simulink library "inp"  (R2021b)
settings: Solver=VariableStepAuto  StartTime=0.0  StopTime=10.0  RelTol=1e-3
undefined symbols (not defined in the file): C_TASK_5MS_S, FALSE, KINP_AcoreReadyToSlp_flg_ovrdflg, KINP_AcoreReadyToSlp_flg_ovrdval, KINP_AllowMovThd_OTA_enum_ovrdflg, KINP_AllowMovThd_OTA_enum_ovrdval, KINP_APSAngleTarget_Deg_ovrdflg, KINP_APSAngleTarget_Deg_ovrdval, KINP_APSDecReq_mps2_ovrdflg, KINP_APSDecReq_mps2_ovrdval, KINP_APSDecReqA_flg_ovrdflg, KINP_APSDecReqA_flg_ovrdval, KINP_APSDFLL_cm_ovrdflg, KINP_APSDFLL_cm_ovrdval, KINP_APSDFLR_cm_ovrdflg, KINP_APSDFLR_cm_ovrdval, KINP_APSDRLL_cm_ovrdflg, KINP_APSDRLL_cm_ovrdval, KINP_APSDRLR_cm_ovrdflg, KINP_APSDRLR_cm_ovrdval, KINP_APSExitCondition_enum_ovrdflg, KINP_APSExitCondition_enum_ovrdval, KINP_APSHWVer_enum_ovrdflg, KINP_APSHWVer_enum_ovrdval, KINP_APSProgressPCT_pct_ovrdflg, KINP_APSProgressPCT_pct_ovrdval, KINP_APSPwrReq_enum_ovrdflg, KINP_APSPwrReq_enum_ovrdval, KINP_APSReq_enum_ovrdflg, KINP_APSReq_enum_ovrdval, KINP_APSRQDisplay_enum_ovrdflg, KINP_APSRQDisplay_enum_ovrdval, KINP_APSRqEPASCtrl_flg_ovrdflg, KINP_APSRqEPASCtrl_flg_ovrdval, KINP_APSShiftPosnReq_enum_ovrdval, KINP_APSShiftPosnReq_enum_ovrflg, KINP_APSSpeedCMD_kph_ovrdval, KINP_APSSpeedCMD_kph_ovrflg, KINP_APSStaSystem_enum_ovrdflg, KINP_APSStaSystem_enum_ovrdval, KINP_APSSWVer_enum_ovrdflg, KINP_APSSWVer_enum_ovrdval, KINP_APSVMCReqA_flg_ovrdval, KINP_APSVMCReqA_flg_ovrflg, KINP_APSVRqEPASCtrl_flg_ovrdflg, KINP_APSVRqEPASCtrl_flg_ovrdval, KINP_AuxBattVolmV_mV_ovrdflg, KINP_AuxBattVolmV_mV_ovrdval, KINP_CAASSta_enum_ovrdflg, KINP_CAASSta_enum_ovrdval, KINP_CAASVMCReqA_flg_ovrdval, KINP_CAASVMCReqA_flg_ovrflg, KINP_CAN1BusOff_flg_ovrdflg, KINP_CAN1BusOff_flg_ovrdval, KINP_CAN2BusOff_flg_ovrdflg, KINP_CAN2BusOff_flg_ovrdval, KINP_CAN3BusOff_flg_ovrdflg, KINP_CAN3BusOff_flg_ovrdval, KINP_CAN4BusOff_flg_ovrdflg, KINP_CAN4BusOff_flg_ovrdval ... (+152)
libraries: FVT_lib x1037, hcu_lib x1
(part 12 of 34)

== system inp/INP/SYS/Subsystem ==
  In1 : Inport
  Constant : Constant  Value=KINP_AuxBattVolmV_mV_ovrdflg
  Constant1 : Constant  Value=KINP_AuxBattVolmV_mV_ovrdval
  Switch : Switch  Criteria=u2 > Threshold
  Out1 : Outport
  wires:
  Constant1/1 -> Switch/1
  Constant/1 -> Switch/2
  In1/1 -> Switch/3
  Switch/1 -> Out1/1

== system inp/INP/SYS/Subsystem1 ==
  In1 : Inport
  Constant : Constant  Value=KINP_NetworkReqCalled_flg_ovrdflg
  Constant1 : Constant  Value=KINP_NetworkReqCalled_flg_ovrdval
  Switch : Switch  Criteria=u2 > Threshold
  Out1 : Outport
  wires:
  Constant1/1 -> Switch/1
  Constant/1 -> Switch/2
  In1/1 -> Switch/3
  Switch/1 -> Out1/1

== system inp/INP/SYS/Subsystem10 ==
  In1 : Inport
  Constant : Constant  Value=KINP_CAN3BusOff_flg_ovrdflg
  Constant1 : Constant  Value=KINP_CAN3BusOff_flg_ovrdval
  Switch : Switch  Criteria=u2 > Threshold
  Out1 : Outport
  wires:
  Constant1/1 -> Switch/1
  Constant/1 -> Switch/2
  In1/1 -> Switch/3
  Switch/1 -> Out1/1

== system inp/INP/SYS/Subsystem11 ==
  In1 : Inport
  Constant : Constant  Value=KINP_CAN6BusOff_flg_ovrdflg
  Constant1 : Constant  Value=KINP_CAN6BusOff_flg_ovrdval
  Switch : Switch  Criteria=u2 > Threshold
  Out1 : Outport
  wires:
  Switch/1 -> Out1/1
  In1/1 -> Switch/3
  Constant/1 -> Switch/2
  Constant1/1 -> Switch/1

== system inp/INP/SYS/Subsystem12 ==
  In1 : Inport
  Constant : Constant  Value=KINP_CAN4BusOff_flg_ovrdflg
  Constant1 : Constant  Value=KINP_CAN4BusOff_flg_ovrdval
  Switch : Switch  Criteria=u2 > Threshold
  Out1 : Outport
  wires:
  Switch/1 -> Out1/1
  In1/1 -> Switch/3
  Constant/1 -> Switch/2
  Constant1/1 -> Switch/1

== system inp/INP/SYS/Subsystem13 ==
  In1 : Inport
  Constant : Constant  Value=KINP_CAN5BusOff_flg_ovrdflg
  Constant1 : Constant  Value=KINP_CAN5BusOff_flg_ovrdval
  Switch : Switch  Criteria=u2 > Threshold
  Out1 : Outport
  wires:
  Constant1/1 -> Switch/1
  Constant/1 -> Switch/2
  In1/1 -> Switch/3
  Switch/1 -> Out1/1

== system inp/INP/SYS/Subsystem2 ==
  In1 : Inport
  Constant : Constant  Value=KINP_Pedal1Ref5V_V_ovrdflg
  Constant1 : Constant  Value=KINP_Pedal1Ref5V_V_ovrdval
  Switch : Switch  Criteria=u2 > Threshold
  Out1 : Outport
  wires:
  Switch/1 -> Out1/1
  In1/1 -> Switch/3
  Constant/1 -> Switch/2
  Constant1/1 -> Switch/1

== system inp/INP/SYS/Subsystem3 ==
  In1 : Inport
  Constant : Constant  Value=KINP_Pedal2Ref5V_V_ovrdflg
  Constant1 : Constant  Value=KINP_Pedal2Ref5V_V_ovrdval
  Switch : Switch  Criteria=u2 > Threshold
  Out1 : Outport
  wires:
  Constant1/1 -> Switch/1
  Constant/1 -> Switch/2
  In1/1 -> Switch/3
  Switch/1 -> Out1/1

== system inp/INP/SYS/Subsystem4 ==
  In1 : Inport
  Constant : Constant  Value=KINP_PwrReq_OTA_enum_ovrdval
  Constant1 : Constant  Value=KINP_PwrReq_OTA_enum_ovrdflg
  Switch : Switch  Criteria=u2 ~= 0
  Out1 : Outport
  wires:
  Constant1/1 -> Switch/2
  Constant/1 -> Switch/1
  In1/1 -> Switch/3
  Switch/1 -> Out1/1

== system inp/INP/SYS/Subsystem5 ==
  In1 : Inport
  Constant : Constant  Value=KINP_AllowMovThd_OTA_enum_ovrdval
  Constant1 : Constant  Value=KINP_AllowMovThd_OTA_enum_ovrdflg
  Switch : Switch  Criteria=u2 ~= 0
  Out1 : Outport
  wires:
  Switch/1 -> Out1/1
  In1/1 -> Switch/3
  Constant/1 -> Switch/1
  Constant1/1 -> Switch/2

== system inp/INP/SYS/Subsystem6 ==
  In1 : Inport
  Constant : Constant  Value=KINP_EvccAplusPwrUpReq_flg_ovrdval
  Constant1 : Constant  Value=KINP_EvccAplusPwrUpReq_flg_ovrdflg
  Switch : Switch  Criteria=u2 ~= 0
  Out1 : Outport
  wires:
  Constant1/1 -> Switch/2
  Constant/1 -> Switch/1
  In1/1 -> Switch/3
  Switch/1 -> Out1/1

== system inp/INP/SYS/Subsystem7 ==
  In1 : Inport
  Constant : Constant  Value=KINP_AcoreReadyToSlp_flg_ovrdval
  Constant1 : Constant  Value=KINP_AcoreReadyToSlp_flg_ovrdflg
  Switch : Switch  Criteria=u2 ~= 0
  Out1 : Outport
  wires:
  Switch/1 -> Out1/1
  In1/1 -> Switch/3
  Constant/1 -> Switch/1
  Constant1/1 -> Switch/2

== system inp/INP/SYS/Subsystem8 ==
  In1 : Inport
  Constant : Constant  Value=KINP_CAN1BusOff_flg_ovrdflg
  Constant1 : Constant  Value=KINP_CAN1BusOff_flg_ovrdval
  Switch : Switch  Criteria=u2 > Threshold
  Out1 : Outport
  wires:
  Constant1/1 -> Switch/1
  Constant/1 -> Switch/2
  In1/1 -> Switch/3
  Switch/1 -> Out1/1

== system inp/INP/SYS/Subsystem9 ==
  In1 : Inport
  Constant : Constant  Value=KINP_CAN2BusOff_flg_ovrdflg
  Constant1 : Constant  Value=KINP_CAN2BusOff_flg_ovrdval
  Switch : Switch  Criteria=u2 > Threshold
  Out1 : Outport
  wires:
  Switch/1 -> Out1/1
  In1/1 -> Switch/3
  Constant/1 -> Switch/2
  Constant1/1 -> Switch/1

== system inp/INP/TPMS/Subsystem ==
  In1 : Inport
  Constant : Constant  Value=KINP_TPMSDataIn_flg_ovrdval
  Constant1 : Constant  Value=KINP_TPMSDataIn_flg_ovrdflg
  Switch : Switch  Criteria=u2 ~= 0
  Out1 : Outport
  wires:
  Switch/1 -> Out1/1
  In1/1 -> Switch/3
  Constant/1 -> Switch/1
  Constant1/1 -> Switch/2

== system inp/INP/TPMS/Subsystem1 ==
  In1 : Inport
  Constant : Constant  Value=KINP_TPMSID_raw_ovrdflg
  Constant1 : Constant  Value=KINP_TPMSID_raw_ovrdval
  Switch : Switch  Criteria=u2 ~= 0
  Out1 : Outport
  wires:
  Constant/1 -> Switch/2
  Constant1/1 -> Switch/1
  Switch/1 -> Out1/1
  In1/1 -> Switch/3

== system inp/INP/TPMS/Subsystem10 ==
  In1 : Inport
  Constant : Constant  Value=KINP_TPMSStorge_flg_ovrflg
  Constant1 : Constant  Value=KINP_TPMSStorge_flg_ovrdval
  Switch : Switch  Criteria=u2 ~= 0
  Out1 : Outport
  wires:
  Constant1/1 -> Switch/1
  Constant/1 -> Switch/2
  In1/1 -> Switch/3
  Switch/1 -> Out1/1

== system inp/INP/TPMS/Subsystem11 ==
  In1 : Inport
  Constant : Constant  Value=KINP_LFID_raw_ovrflg
  Constant1 : Constant  Value=KINP_LFID_raw_ovrdval
  Switch : Switch  Criteria=u2 ~= 0
  Out1 : Outport
  wires:
  Switch/1 -> Out1/1
  In1/1 -> Switch/3
  Constant/1 -> Switch/2
  Constant1/1 -> Switch/1

== system inp/INP/TPMS/Subsystem12 ==
  In1 : Inport
  Constant : Constant  Value=KINP_RFID_raw_ovrdval
  Constant1 : Constant  Value=KINP_RFID_raw_ovrdval
  Switch : Switch  Criteria=u2 ~= 0
  Out1 : Outport
  wires:
  Constant1/1 -> Switch/1
  Constant/1 -> Switch/2
  In1/1 -> Switch/3
  Switch/1 -> Out1/1

== system inp/INP/TPMS/Subsystem13 ==
  In1 : Inport
  Constant : Constant  Value=KINP_LRID_raw_ovrdval
  Constant1 : Constant  Value=KINP_LRID_raw_ovrdval
  Switch : Switch  Criteria=u2 ~= 0
  Out1 : Outport
  wires:
  Switch/1 -> Out1/1
  In1/1 -> Switch/3
  Constant/1 -> Switch/2
  Constant1/1 -> Switch/1

== system inp/INP/TPMS/Subsystem14 ==
  In1 : Inport
  Constant : Constant  Value=KINP_RRID_raw_ovrdval
  Constant1 : Constant  Value=KINP_RRID_raw_ovrdval
  Switch : Switch  Criteria=u2 ~= 0
  Out1 : Outport
  wires:
  Constant1/1 -> Switch/1
  Constant/1 -> Switch/2
  In1/1 -> Switch/3
  Switch/1 -> Out1/1

== system inp/INP/TPMS/Subsystem2 ==
  In1 : Inport
  Constant : Constant  Value=KINP_TPMSPressure_raw_ovrdflg
  Constant1 : Constant  Value=KINP_TPMSPressure_raw_ovrdval
  Switch : Switch  Criteria=u2 ~= 0
  Out1 : Outport
  wires:
  Constant/1 -> Switch/2
  Constant1/1 -> Switch/1
  Switch/1 -> Out1/1
  In1/1 -> Switch/3

== system inp/INP/TPMS/Subsystem3 ==
  In1 : Inport
  Constant : Constant  Value=KINP_TPMSTemp_raw_ovrdflg
  Constant1 : Constant  Value=KINP_TPMSTemp_raw_ovrdval
  Switch : Switch  Criteria=u2 ~= 0
  Out1 : Outport
  wires:
  Constant/1 -> Switch/2
  Constant1/1 -> Switch/1
  Switch/1 -> Out1/1
  In1/1 -> Switch/3

== system inp/INP/TPMS/Subsystem4 ==
  In1 : Inport
  Constant : Constant  Value=KINP_TPMSSta_enum_ovrdflg
  Constant1 : Constant  Value=KINP_TPMSSta_enum_ovrdval
  Switch : Switch  Criteria=u2 ~= 0
  Out1 : Outport
  wires:
  Constant/1 -> Switch/2
  Constant1/1 -> Switch/1
  Switch/1 -> Out1/1
  In1/1 -> Switch/3

== system inp/INP/TPMS/Subsystem5 ==
  In1 : Inport
  Constant : Constant  Value=KINP_TPMSPressureMi_raw_ovrdflg
  Constant1 : Constant  Value=KINP_TPMSPressureMi_raw_ovrdval
  Switch : Switch  Criteria=u2 ~= 0
  Out1 : Outport
  wires:
  Constant/1 -> Switch/2
  Constant1/1 -> Switch/1
  Switch/1 -> Out1/1
  In1/1 -> Switch/3

== system inp/INP/TPMS/Subsystem6 ==
  In1 : Inport
  Constant : Constant  Value=KINP_TPMSCRC_crc_ovrdflg
  Constant1 : Constant  Value=KINP_TPMSCRC_crc_ovrdval
  Switch : Switch  Criteria=u2 ~= 0
  Out1 : Outport
  wires:
  Constant/1 -> Switch/2
  Constant1/1 -> Switch/1
  Switch/1 -> Out1/1
  In1/1 -> Switch/3

== system inp/INP/TPMS/Subsystem7 ==
  In1 : Inport
  Constant : Constant  Value=KINP_TPMSCRCCalc_crc_ovrdflg
  Constant1 : Constant  Value=KINP_TPMSCRCCalc_crc_ovrdval
  Switch : Switch  Criteria=u2 ~= 0
  Out1 : Outport
  wires:
  Constant/1 -> Switch/2
  Constant1/1 -> Switch/1
  Switch/1 -> Out1/1
  In1/1 -> Switch/3

== system inp/INP/TPMS/Subsystem8 ==
  In1 : Inport
  Constant : Constant  Value=KINP_TPMSFAT_flg_ovrflg
  Constant1 : Constant  Value=KINP_TPMSFAT_flg_ovrdval
  Switch : Switch  Criteria=u2 ~= 0
  Out1 : Outport
  wires:
  Switch/1 -> Out1/1
  In1/1 -> Switch/3
  Constant1/1 -> Switch/1
  Constant/1 -> Switch/2

== system inp/INP/TPMS/Subsystem9 ==
  In1 : Inport
  Constant : Constant  Value=KINP_TPMSBattLow_flg_ovrflg
  Constant1 : Constant  Value=KINP_TPMSBattLow_flg_ovrdval
  Switch : Switch  Criteria=u2 ~= 0
  Out1 : Outport
  wires:
  Switch/1 -> Out1/1
  In1/1 -> Switch/3
  Constant/1 -> Switch/2
  Constant1/1 -> Switch/1

== system inp/INP/CAN1/SignalCheck/ABM1 ==
  BHAL_outputs : Inport
  inp_CanValid_bus : Inport  Port=2
  ABM1CSErr : FVT_lib/inp/can_signal_template  SystemSampleTime=-1  VariantActivationTime=update diagram  Latency=0  AutoFrameSizeCalculation=off
      link override defval: Value=KINP_ABM1CSErr_flg_defval
      link override ovrdflg: Value=KINP_ABM1CSErr_flg_ovrdflg
      link override ovrdval: Value=KINP_ABM1CSErr_flg_ovrdval
  ABM1RCErr : FVT_lib/inp/can_signal_template  SystemSampleTime=-1  VariantActivationTime=update diagram  Latency=0  AutoFrameSizeCalculation=off
      link override defval: Value=KINP_ABM1RCErr_flg_defval
      link override ovrdflg: Value=KINP_ABM1RCErr_flg_ovrdflg
      link override ovrdval: Value=KINP_ABM1RCErr_flg_ovrdval
  ABMPassengerODSSta : FVT_lib/inp/can_signal_template  SystemSampleTime=-1  VariantActivationTime=update diagram  Latency=0  AutoFrameSizeCalculation=off
      link override defval: Value=KINP_ABMPassengerODSSta_flg_defval
      link override ovrdflg: Value=KINP_ABMPassengerODSSta_flg_ovrdflg
      link override ovrdval: Value=KINP_ABMPassengerODSSta_flg_ovrdval
  ABMRearPassengerCTRODSSta : FVT_lib/inp/can_signal_template  SystemSampleTime=-1  VariantActivationTime=update diagram  Latency=0  AutoFrameSizeCalculation=off
      link override defval: Value=KINP_ABMRearPassengerCTRODSSta_flg_defval
      link override ovrdflg: Value=KINP_ABMRearPassengerCTRODSSta_flg_ovrdflg
      link override ovrdval: Value=KINP_ABMRearPassengerCTRODSSta_flg_ovrdval
  ABMRearPassengerLHODSSta : FVT_lib/inp/can_signal_template  SystemSampleTime=-1  VariantActivationTime=update diagram  Latency=0  AutoFrameSizeCalculation=off
      link override defval: Value=KINP_ABMRearPassengerLHODSSta_flg_defval
      link override ovrdflg: Value=KINP_ABMRearPassengerLHODSSta_flg_ovrdflg
      link override ovrdval: Value=KINP_ABMRearPassengerLHODSSta_flg_ovrdval
  ABMRearPassengerRHODSSta : FVT_lib/inp/can_signal_template  SystemSampleTime=-1  VariantActivationTime=update diagram  Latency=0  AutoFrameSizeCalculation=off
      link override defval: Value=KINP_ABMRearPassengerRHODSSta_flg_defval
      link override ovrdflg: Value=KINP_ABMRearPassengerRHODSSta_flg_ovrdflg
      link override ovrdval: Value=KINP_ABMRearPassengerRHODSSta_flg_ovrdval
  AirBagFailCmd : FVT_lib/inp/can_signal_template  SystemSampleTime=-1  VariantActivationTime=update diagram  Latency=0  AutoFrameSizeCalculation=off
      link override defval: Value=KINP_AirBagFailCmd_flg_defval
      link override ovrdflg: Value=KINP_AirBagFailCmd_flg_ovrdflg
      link override ovrdval: Value=KINP_AirBagFailCmd_flg_ovrdval
  ChecksumABM1 : FVT_lib/inp/can_signal_template  SystemSampleTime=-1  VariantActivationTime=update diagram  Latency=0  AutoFrameSizeCalculation=off
      link override defval: Value=KINP_ChecksumABM1_enum_defval
      link override ovrdflg: Value=KINP_ChecksumABM1_enum_ovrdflg
      link override ovrdval: Value=KINP_ChecksumABM1_enum_ovrdval
  CrashOutputSts : FVT_lib/inp/can_signal_template  SystemSampleTime=-1  VariantActivationTime=update diagram  Latency=0  AutoFrameSizeCalculation=off
      link override defval: Value=KINP_CrashOutputSts_enum_defval
      link override ovrdflg: Value=KINP_CrashOutputSts_enum_ovrdflg
      link override ovrdval: Value=KINP_CrashOutputSts_enum_ovrdval
  DriverSeatBeltCmd : FVT_lib/inp/can_signal_template  SystemSampleTime=-1  VariantActivationTime=update diagram  Latency=0  AutoFrameSizeCalculation=off
      link override defval: Value=KINP_DriverSeatBeltCmd_flg_defval
      link override ovrdflg: Value=KINP_DriverSeatBeltCmd_flg_ovrdflg
      link override ovrdval: Value=KINP_DriverSeatBeltCmd_flg_ovrdval
  LifeCountABM1 : FVT_lib/inp/can_signal_template  SystemSampleTime=-1  VariantActivationTime=update diagram  Latency=0  AutoFrameSizeCalculation=off
      link override defval: Value=KINP_LifeCountABM1_enum_defval
      link override ovrdflg: Value=KINP_LifeCountABM1_enum_ovrdflg
      link override ovrdval: Value=KINP_LifeCountABM1_enum_ovrdval
  PABSwitchCmd : FVT_lib/inp/can_signal_template  SystemSampleTime=-1  VariantActivationTime=update diagram  Latency=0  AutoFrameSizeCalculation=off
      link override defval: Value=KINP_PABSwitchCmd_flg_defval
      link override ovrdflg: Value=KINP_PABSwitchCmd_flg_ovrdflg
      link override ovrdval: Value=KINP_PABSwitchCmd_flg_ovrdval
  PsngrSeatBeltCmd : FVT_lib/inp/can_signal_template  SystemSampleTime=-1  VariantActivationTime=update diagram  Latency=0  AutoFrameSizeCalculation=off
      link override defval: Value=KINP_PsngrSeatBeltCmd_flg_defval
      link override ovrdflg: Value=KINP_PsngrSeatBeltCmd_flg_ovrdflg
      link override ovrdval: Value=KINP_PsngrSeatBeltCmd_flg_ovrdval
  RCenterSeatBeltCmd : FVT_lib/inp/can_signal_template  SystemSampleTime=-1  VariantActivationTime=update diagram  Latency=0  AutoFrameSizeCalculation=off
      link override defval: Value=KINP_RCenterSeatBeltCmd_flg_defval
      link override ovrdflg: Value=KINP_RCenterSeatBeltCmd_flg_ovrdflg
      link override ovrdval: Value=KINP_RCenterSeatBeltCmd_flg_ovrdval
  RDriverSeatBeltCmd : FVT_lib/inp/can_signal_template  SystemSampleTime=-1  VariantActivationTime=update diagram  Latency=0  AutoFrameSizeCalculation=off
      link override defval: Value=KINP_RDriverSeatBeltCmd_flg_defval
      link override ovrdflg: Value=KINP_RDriverSeatBeltCmd_flg_ovrdflg
      link override ovrdval: Value=KINP_RDriverSeatBeltCmd_flg_ovrdval
  RPsngrSeatBeltCmd : FVT_lib/inp/can_signal_template  SystemSampleTime=-1  VariantActivationTime=update diagram  Latency=0  AutoFrameSizeCalculation=off
      link override defval: Value=KINP_RPsngrSeatBeltCmd_flg_defval
      link override ovrdflg: Value=KINP_RPsngrSeatBeltCmd_flg_ovrdflg
      link override ovrdval: Value=KINP_RPsngrSeatBeltCmd_flg_ovrdval
  TLHPsngrSeatBeltCmd : FVT_lib/inp/can_signal_template  SystemSampleTime=-1  VariantActivationTime=update diagram  Latency=0  AutoFrameSizeCalculation=off
      link override defval: Value=KINP_TLHPsngrSeatBeltCmd_flg_defval
      link override ovrdflg: Value=KINP_TLHPsngrSeatBeltCmd_flg_ovrdflg
      link override ovrdval: Value=KINP_TLHPsngrSeatBeltCmd_flg_ovrdval
  TRHPsngrSeatBeltCmd : FVT_lib/inp/can_signal_template  SystemSampleTime=-1  VariantActivationTime=update diagram  Latency=0  AutoFrameSizeCalculation=off
      link override defval: Value=KINP_TRHPsngrSeatBeltCmd_flg_defval
      link override ovrdflg: Value=KINP_TRHPsngrSeatBeltCmd_flg_ovrdflg
      link override ovrdval: Value=KINP_TRHPsngrSeatBeltCmd_flg_ovrdval
  Terminator_{1..18} (18 alike) : Terminator
  True_VHAL_ABM1CSErr_flg : Constant  Value=TRUE  OutDataTypeStr=boolean
  True_VHAL_ABM1RCErr_flg : Constant  Value=TRUE  OutDataTypeStr=boolean
  True_VHAL_ABMPassengerODSSta_flg : Constant  Value=TRUE  OutDataTypeStr=boolean
  True_VHAL_ABMRearPassengerCTRODSSta_flg : Constant  Value=TRUE  OutDataTypeStr=boolean
  True_VHAL_ABMRearPassengerLHODSSta_flg : Constant  Value=TRUE  OutDataTypeStr=boolean
  True_VHAL_ABMRearPassengerRHODSSta_flg : Constant  Value=TRUE  OutDataTypeStr=boolean
  True_VHAL_AirBagFailCmd_flg : Constant  Value=TRUE  OutDataTypeStr=boolean
  True_VHAL_ChecksumABM1_enum : Constant  Value=TRUE  OutDataTypeStr=boolean
  True_VHAL_CrashOutputSts_enum : Constant  Value=TRUE  OutDataTypeStr=boolean
  True_VHAL_DriverSeatBeltCmd_flg : Constant  Value=TRUE  OutDataTypeStr=boolean
  True_VHAL_LifeCountABM1_enum : Constant  Value=TRUE  OutDataTypeStr=boolean
  True_VHAL_PABSwitchCmd_flg : Constant  Value=TRUE  OutDataTypeStr=boolean
  True_VHAL_PsngrSeatBeltCmd_flg : Constant  Value=TRUE  OutDataTypeStr=boolean
  True_VHAL_RCenterSeatBeltCmd_flg : Constant  Value=TRUE  OutDataTypeStr=boolean
  True_VHAL_RDriverSeatBeltCmd_flg : Constant  Value=TRUE  OutDataTypeStr=boolean
  True_VHAL_RPsngrSeatBeltCmd_flg : Constant  Value=TRUE  OutDataTypeStr=boolean
  True_VHAL_TLHPsngrSeatBeltCmd_flg : Constant  Value=TRUE  OutDataTypeStr=boolean
  True_VHAL_TRHPsngrSeatBeltCmd_flg : Constant  Value=TRUE  OutDataTypeStr=boolean
  slr1_{1..18} (18 alike) : BusSelector  OutputSignals=VINP_CANMsgValidABM1_flg
  slr_VHAL_ABM1CSErr_flg : BusSelector  OutputSignals=VHAL_ABM1CSErr_flg
  slr_VHAL_ABM1RCErr_flg : BusSelector  OutputSignals=VHAL_ABM1RCErr_flg
  slr_VHAL_ABMPassengerODSSta_flg : BusSelector  OutputSignals=VHAL_ABMPassengerODSSta_flg
  slr_VHAL_ABMRearPassengerCTRODSSta_flg : BusSelector  OutputSignals=VHAL_ABMRearPassengerCTRODSSta_flg
  slr_VHAL_ABMRearPassengerLHODSSta_flg : BusSelector  OutputSignals=VHAL_ABMRearPassengerLHODSSta_flg
  slr_VHAL_ABMRearPassengerRHODSSta_flg : BusSelector  OutputSignals=VHAL_ABMRearPassengerRHODSSta_flg
  slr_VHAL_AirBagFailCmd_flg : BusSelector  OutputSignals=VHAL_AirBagFailCmd_flg
  slr_VHAL_ChecksumABM1_enum : BusSelector  OutputSignals=VHAL_ChecksumABM1_enum
  slr_VHAL_CrashOutputSts_enum : BusSelector  OutputSignals=VHAL_CrashOutputSts_enum
  slr_VHAL_DriverSeatBeltCmd_flg : BusSelector  OutputSignals=VHAL_DriverSeatBeltCmd_flg
  slr_VHAL_LifeCountABM1_enum : BusSelector  OutputSignals=VHAL_LifeCountABM1_enum
  slr_VHAL_PABSwitchCmd_flg : BusSelector  OutputSignals=VHAL_PABSwitchCmd_flg
  slr_VHAL_PsngrSeatBeltCmd_flg : BusSelector  OutputSignals=VHAL_PsngrSeatBeltCmd_flg
  slr_VHAL_RCenterSeatBeltCmd_flg : BusSelector  OutputSignals=VHAL_RCenterSeatBeltCmd_flg
  slr_VHAL_RDriverSeatBeltCmd_flg : BusSelector  OutputSignals=VHAL_RDriverSeatBeltCmd_flg
  slr_VHAL_RPsngrSeatBeltCmd_flg : BusSelector  OutputSignals=VHAL_RPsngrSeatBeltCmd_flg
  slr_VHAL_TLHPsngrSeatBeltCmd_flg : BusSelector  OutputSignals=VHAL_TLHPsngrSeatBeltCmd_flg
  slr_VHAL_TRHPsngrSeatBeltCmd_flg : BusSelector  OutputSignals=VHAL_TRHPsngrSeatBeltCmd_flg
  VINP_ABM1CSErr_flg : Outport
  VINP_ABM1RCErr_flg : Outport  Port=2
  VINP_ABMPassengerODSSta_flg : Outport  Port=3
  VINP_ABMRearPassengerCTRODSSta_flg : Outport  Port=4
  VINP_ABMRearPassengerLHODSSta_flg : Outport  Port=5
  VINP_ABMRearPassengerRHODSSta_flg : Outport  Port=6
  VINP_AirBagFailCmd_flg : Outport  Port=7
  VINP_ChecksumABM1_enum : Outport  Port=8
  VINP_CrashOutputSts_enum : Outport  Port=9
  VINP_DriverSeatBeltCmd_flg : Outport  Port=10
  VINP_LifeCountABM1_enum : Outport  Port=11
  VINP_PABSwitchCmd_flg : Outport  Port=12
  VINP_PsngrSeatBeltCmd_flg : Outport  Port=13
  VINP_RCenterSeatBeltCmd_flg : Outport  Port=14
  VINP_RDriverSeatBeltCmd_flg : Outport  Port=15
  VINP_RPsngrSeatBeltCmd_flg : Outport  Port=16
  VINP_TLHPsngrSeatBeltCmd_flg : Outport  Port=17
  VINP_TRHPsngrSeatBeltCmd_flg : Outport  Port=18
  wires:
  BHAL_outputs/1 -> [BHAL_outputs]
  inp_CanValid_bus/1 -> [inp_CanValid_bus]
  [BHAL_outputs] -> slr_VHAL_ABM1CSErr_flg/1
  slr_VHAL_ABM1CSErr_flg/1 -> ABM1CSErr/1  "<VHAL_ABM1CSErr_flg>"
  True_VHAL_ABM1CSErr_flg/1 -> ABM1CSErr/2
  [inp_CanValid_bus] -> slr1_1/1
  slr1_1/1 -> ABM1CSErr/3  "<VINP_CANMsgValidABM1_flg>"
  ABM1CSErr/1 -> VINP_ABM1CSErr_flg/1  "VINP_ABM1CSErr_flg"
  ABM1CSErr/2 -> Terminator_1/1
  [BHAL_outputs] -> slr_VHAL_ABM1RCErr_flg/1
  slr_VHAL_ABM1RCErr_flg/1 -> ABM1RCErr/1  "<VHAL_ABM1RCErr_flg>"
  True_VHAL_ABM1RCErr_flg/1 -> ABM1RCErr/2
  [inp_CanValid_bus] -> slr1_2/1
  slr1_2/1 -> ABM1RCErr/3  "<VINP_CANMsgValidABM1_flg>"
  ABM1RCErr/1 -> VINP_ABM1RCErr_flg/1  "VINP_ABM1RCErr_flg"
  ABM1RCErr/2 -> Terminator_2/1
  [BHAL_outputs] -> slr_VHAL_ABMPassengerODSSta_flg/1
  slr_VHAL_ABMPassengerODSSta_flg/1 -> ABMPassengerODSSta/1  "<VHAL_ABMPassengerODSSta_flg>"
  True_VHAL_ABMPassengerODSSta_flg/1 -> ABMPassengerODSSta/2
  [inp_CanValid_bus] -> slr1_3/1
  slr1_3/1 -> ABMPassengerODSSta/3  "<VINP_CANMsgValidABM1_flg>"
  ABMPassengerODSSta/1 -> VINP_ABMPassengerODSSta_flg/1  "VINP_ABMPassengerODSSta_flg"
  ABMPassengerODSSta/2 -> Terminator_3/1
  [BHAL_outputs] -> slr_VHAL_ABMRearPassengerCTRODSSta_flg/1
  slr_VHAL_ABMRearPassengerCTRODSSta_flg/1 -> ABMRearPassengerCTRODSSta/1  "<VHAL_ABMRearPassengerCTRODSSta_flg>"
  True_VHAL_ABMRearPassengerCTRODSSta_flg/1 -> ABMRearPassengerCTRODSSta/2
  [inp_CanValid_bus] -> slr1_4/1
  slr1_4/1 -> ABMRearPassengerCTRODSSta/3  "<VINP_CANMsgValidABM1_flg>"
  ABMRearPassengerCTRODSSta/1 -> VINP_ABMRearPassengerCTRODSSta_flg/1  "VINP_ABMRearPassengerCTRODSSta_flg"
  ABMRearPassengerCTRODSSta/2 -> Terminator_4/1
  [BHAL_outputs] -> slr_VHAL_ABMRearPassengerLHODSSta_flg/1
  slr_VHAL_ABMRearPassengerLHODSSta_flg/1 -> ABMRearPassengerLHODSSta/1  "<VHAL_ABMRearPassengerLHODSSta_flg>"
  True_VHAL_ABMRearPassengerLHODSSta_flg/1 -> ABMRearPassengerLHODSSta/2
  [inp_CanValid_bus] -> slr1_5/1
  slr1_5/1 -> ABMRearPassengerLHODSSta/3  "<VINP_CANMsgValidABM1_flg>"
  ABMRearPassengerLHODSSta/1 -> VINP_ABMRearPassengerLHODSSta_flg/1  "VINP_ABMRearPassengerLHODSSta_flg"
  ABMRearPassengerLHODSSta/2 -> Terminator_5/1
  [BHAL_outputs] -> slr_VHAL_ABMRearPassengerRHODSSta_flg/1
  slr_VHAL_ABMRearPassengerRHODSSta_flg/1 -> ABMRearPassengerRHODSSta/1  "<VHAL_ABMRearPassengerRHODSSta_flg>"
  True_VHAL_ABMRearPassengerRHODSSta_flg/1 -> ABMRearPassengerRHODSSta/2
  [inp_CanValid_bus] -> slr1_6/1
  slr1_6/1 -> ABMRearPassengerRHODSSta/3  "<VINP_CANMsgValidABM1_flg>"
  ABMRearPassengerRHODSSta/1 -> VINP_ABMRearPassengerRHODSSta_flg/1  "VINP_ABMRearPassengerRHODSSta_flg"
  ABMRearPassengerRHODSSta/2 -> Terminator_6/1
  [BHAL_outputs] -> slr_VHAL_AirBagFailCmd_flg/1
  slr_VHAL_AirBagFailCmd_flg/1 -> AirBagFailCmd/1  "<VHAL_AirBagFailCmd_flg>"
  True_VHAL_AirBagFailCmd_flg/1 -> AirBagFailCmd/2
  [inp_CanValid_bus] -> slr1_7/1
  slr1_7/1 -> AirBagFailCmd/3  "<VINP_CANMsgValidABM1_flg>"
  AirBagFailCmd/1 -> VINP_AirBagFailCmd_flg/1  "VINP_AirBagFailCmd_flg"
  AirBagFailCmd/2 -> Terminator_7/1
  [BHAL_outputs] -> slr_VHAL_ChecksumABM1_enum/1
  slr_VHAL_ChecksumABM1_enum/1 -> ChecksumABM1/1  "<VHAL_ChecksumABM1_enum>"
  True_VHAL_ChecksumABM1_enum/1 -> ChecksumABM1/2
  [inp_CanValid_bus] -> slr1_8/1
  slr1_8/1 -> ChecksumABM1/3  "<VINP_CANMsgValidABM1_flg>"
  ChecksumABM1/1 -> VINP_ChecksumABM1_enum/1  "VINP_ChecksumABM1_enum"
  ChecksumABM1/2 -> Terminator_8/1
  [BHAL_outputs] -> slr_VHAL_CrashOutputSts_enum/1
  slr_VHAL_CrashOutputSts_enum/1 -> CrashOutputSts/1  "<VHAL_CrashOutputSts_enum>"
  True_VHAL_CrashOutputSts_enum/1 -> CrashOutputSts/2
  [inp_CanValid_bus] -> slr1_9/1
  slr1_9/1 -> CrashOutputSts/3  "<VINP_CANMsgValidABM1_flg>"
  CrashOutputSts/1 -> VINP_CrashOutputSts_enum/1  "VINP_CrashOutputSts_enum"
  CrashOutputSts/2 -> Terminator_9/1
  [BHAL_outputs] -> slr_VHAL_DriverSeatBeltCmd_flg/1
  slr_VHAL_DriverSeatBeltCmd_flg/1 -> DriverSeatBeltCmd/1  "<VHAL_DriverSeatBeltCmd_flg>"
  True_VHAL_DriverSeatBeltCmd_flg/1 -> DriverSeatBeltCmd/2
  [inp_CanValid_bus] -> slr1_10/1
  slr1_10/1 -> DriverSeatBeltCmd/3  "<VINP_CANMsgValidABM1_flg>"
  DriverSeatBeltCmd/1 -> VINP_DriverSeatBeltCmd_flg/1  "VINP_DriverSeatBeltCmd_flg"
  DriverSeatBeltCmd/2 -> Terminator_10/1
  [BHAL_outputs] -> slr_VHAL_LifeCountABM1_enum/1
  slr_VHAL_LifeCountABM1_enum/1 -> LifeCountABM1/1  "<VHAL_LifeCountABM1_enum>"
  True_VHAL_LifeCountABM1_enum/1 -> LifeCountABM1/2
  [inp_CanValid_bus] -> slr1_11/1
  slr1_11/1 -> LifeCountABM1/3  "<VINP_CANMsgValidABM1_flg>"
  LifeCountABM1/1 -> VINP_LifeCountABM1_enum/1  "VINP_LifeCountABM1_enum"
  LifeCountABM1/2 -> Terminator_11/1
  [BHAL_outputs] -> slr_VHAL_PABSwitchCmd_flg/1
  slr_VHAL_PABSwitchCmd_flg/1 -> PABSwitchCmd/1  "<VHAL_PABSwitchCmd_flg>"
  True_VHAL_PABSwitchCmd_flg/1 -> PABSwitchCmd/2
  [inp_CanValid_bus] -> slr1_12/1
  slr1_12/1 -> PABSwitchCmd/3  "<VINP_CANMsgValidABM1_flg>"
  PABSwitchCmd/1 -> VINP_PABSwitchCmd_flg/1  "VINP_PABSwitchCmd_flg"
  PABSwitchCmd/2 -> Terminator_12/1
  [BHAL_outputs] -> slr_VHAL_PsngrSeatBeltCmd_flg/1
  slr_VHAL_PsngrSeatBeltCmd_flg/1 -> PsngrSeatBeltCmd/1  "<VHAL_PsngrSeatBeltCmd_flg>"
  True_VHAL_PsngrSeatBeltCmd_flg/1 -> PsngrSeatBeltCmd/2
  [inp_CanValid_bus] -> slr1_13/1
  slr1_13/1 -> PsngrSeatBeltCmd/3  "<VINP_CANMsgValidABM1_flg>"
  PsngrSeatBeltCmd/1 -> VINP_PsngrSeatBeltCmd_flg/1  "VINP_PsngrSeatBeltCmd_flg"
  PsngrSeatBeltCmd/2 -> Terminator_13/1
  [BHAL_outputs] -> slr_VHAL_RCenterSeatBeltCmd_flg/1
  slr_VHAL_RCenterSeatBeltCmd_flg/1 -> RCenterSeatBeltCmd/1  "<VHAL_RCenterSeatBeltCmd_flg>"
  True_VHAL_RCenterSeatBeltCmd_flg/1 -> RCenterSeatBeltCmd/2
  [inp_CanValid_bus] -> slr1_14/1
  slr1_14/1 -> RCenterSeatBeltCmd/3  "<VINP_CANMsgValidABM1_flg>"
  RCenterSeatBeltCmd/1 -> VINP_RCenterSeatBeltCmd_flg/1  "VINP_RCenterSeatBeltCmd_flg"
  RCenterSeatBeltCmd/2 -> Terminator_14/1
  [BHAL_outputs] -> slr_VHAL_RDriverSeatBeltCmd_flg/1
  slr_VHAL_RDriverSeatBeltCmd_flg/1 -> RDriverSeatBeltCmd/1  "<VHAL_RDriverSeatBeltCmd_flg>"
  True_VHAL_RDriverSeatBeltCmd_flg/1 -> RDriverSeatBeltCmd/2
  [inp_CanValid_bus] -> slr1_15/1
  slr1_15/1 -> RDriverSeatBeltCmd/3  "<VINP_CANMsgValidABM1_flg>"
  RDriverSeatBeltCmd/1 -> VINP_RDriverSeatBeltCmd_flg/1  "VINP_RDriverSeatBeltCmd_flg"
  RDriverSeatBeltCmd/2 -> Terminator_15/1
  [BHAL_outputs] -> slr_VHAL_RPsngrSeatBeltCmd_flg/1
  slr_VHAL_RPsngrSeatBeltCmd_flg/1 -> RPsngrSeatBeltCmd/1  "<VHAL_RPsngrSeatBeltCmd_flg>"
  True_VHAL_RPsngrSeatBeltCmd_flg/1 -> RPsngrSeatBeltCmd/2
  [inp_CanValid_bus] -> slr1_16/1
  slr1_16/1 -> RPsngrSeatBeltCmd/3  "<VINP_CANMsgValidABM1_flg>"
  RPsngrSeatBeltCmd/1 -> VINP_RPsngrSeatBeltCmd_flg/1  "VINP_RPsngrSeatBeltCmd_flg"
  RPsngrSeatBeltCmd/2 -> Terminator_16/1
  [BHAL_outputs] -> slr_VHAL_TLHPsngrSeatBeltCmd_flg/1
  slr_VHAL_TLHPsngrSeatBeltCmd_flg/1 -> TLHPsngrSeatBeltCmd/1  "<VHAL_TLHPsngrSeatBeltCmd_flg>"
  True_VHAL_TLHPsngrSeatBeltCmd_flg/1 -> TLHPsngrSeatBeltCmd/2
  [inp_CanValid_bus] -> slr1_17/1
  slr1_17/1 -> TLHPsngrSeatBeltCmd/3  "<VINP_CANMsgValidABM1_flg>"
  TLHPsngrSeatBeltCmd/1 -> VINP_TLHPsngrSeatBeltCmd_flg/1  "VINP_TLHPsngrSeatBeltCmd_flg"
  TLHPsngrSeatBeltCmd/2 -> Terminator_17/1
  [BHAL_outputs] -> slr_VHAL_TRHPsngrSeatBeltCmd_flg/1
  slr_VHAL_TRHPsngrSeatBeltCmd_flg/1 -> TRHPsngrSeatBeltCmd/1  "<VHAL_TRHPsngrSeatBeltCmd_flg>"
  True_VHAL_TRHPsngrSeatBeltCmd_flg/1 -> TRHPsngrSeatBeltCmd/2
  [inp_CanValid_bus] -> slr1_18/1
  slr1_18/1 -> TRHPsngrSeatBeltCmd/3  "<VINP_CANMsgValidABM1_flg>"
  TRHPsngrSeatBeltCmd/1 -> VINP_TRHPsngrSeatBeltCmd_flg/1  "VINP_TRHPsngrSeatBeltCmd_flg"
  TRHPsngrSeatBeltCmd/2 -> Terminator_18/1

== system inp/INP/CAN1/SignalCheck/EPB1 ==
  BHAL_outputs : Inport
  inp_CanValid_bus : Inport  Port=2
  DOASta : FVT_lib/inp/can_signal_template  SystemSampleTime=-1  VariantActivationTime=update diagram  Latency=0  AutoFrameSizeCalculation=off
      link override defval: Value=KINP_DOASta_flg_defval
      link override ovrdflg: Value=KINP_DOASta_flg_ovrdflg
      link override ovrdval: Value=KINP_DOASta_flg_ovrdval
  EPB1CSErr : FVT_lib/inp/can_signal_template  SystemSampleTime=-1  VariantActivationTime=update diagram  Latency=0  AutoFrameSizeCalculation=off
      link override defval: Value=KINP_EPB1CSErr_flg_defval
      link override ovrdflg: Value=KINP_EPB1CSErr_flg_ovrdflg
      link override ovrdval: Value=KINP_EPB1CSErr_flg_ovrdval
  EPB1RC : FVT_lib/inp/can_signal_template  SystemSampleTime=-1  VariantActivationTime=update diagram  Latency=0  AutoFrameSizeCalculation=off
      link override defval: Value=KINP_EPB1RC_enum_defval
      link override ovrdflg: Value=KINP_EPB1RC_enum_ovrdflg
      link override ovrdval: Value=KINP_EPB1RC_enum_ovrdval
  EPB1RCErr : FVT_lib/inp/can_signal_template  SystemSampleTime=-1  VariantActivationTime=update diagram  Latency=0  AutoFrameSizeCalculation=off
      link override defval: Value=KINP_EPB1RCErr_flg_defval
      link override ovrdflg: Value=KINP_EPB1RCErr_flg_ovrdflg
      link override ovrdval: Value=KINP_EPB1RCErr_flg_ovrdval
  EPBCarWashMode : FVT_lib/inp/can_signal_template  SystemSampleTime=-1  VariantActivationTime=update diagram  Latency=0  AutoFrameSizeCalculation=off
      link override defval: Value=KINP_EPBCarWashMode_flg_defval
      link override ovrdflg: Value=KINP_EPBCarWashMode_flg_ovrdflg
      link override ovrdval: Value=KINP_EPBCarWashMode_flg_ovrdval
  EPBErrSta : FVT_lib/inp/can_signal_template  SystemSampleTime=-1  VariantActivationTime=update diagram  Latency=0  AutoFrameSizeCalculation=off
      link override defval: Value=KINP_EPBErrSta_enum_defval
      link override ovrdflg: Value=KINP_EPBErrSta_enum_ovrdflg
      link override ovrdval: Value=KINP_EPBErrSta_enum_ovrdval
  EPBExtApplyAvail : FVT_lib/inp/can_signal_template  SystemSampleTime=-1  VariantActivationTime=update diagram  Latency=0  AutoFrameSizeCalculation=off
      link override defval: Value=KINP_EPBExtApplyAvail_flg_defval
      link override ovrdflg: Value=KINP_EPBExtApplyAvail_flg_ovrdflg
      link override ovrdval: Value=KINP_EPBExtApplyAvail_flg_ovrdval
  EPBExtReleaseAvail : FVT_lib/inp/can_signal_template  SystemSampleTime=-1  VariantActivationTime=update diagram  Latency=0  AutoFrameSizeCalculation=off
      link override defval: Value=KINP_EPBExtReleaseAvail_flg_defval
      link override ovrdflg: Value=KINP_EPBExtReleaseAvail_flg_ovrdflg
      link override ovrdval: Value=KINP_EPBExtReleaseAvail_flg_ovrdval
  EPBSta : FVT_lib/inp/can_signal_template  SystemSampleTime=-1  VariantActivationTime=update diagram  Latency=0  AutoFrameSizeCalculation=off
      link override defval: Value=KINP_EPBSta_enum_defval
      link override ovrdflg: Value=KINP_EPBSta_enum_ovrdflg
      link override ovrdval: Value=KINP_EPBSta_enum_ovrdval
  Terminator_{1..9} (9 alike) : Terminator
  True_VHAL_DOASta_flg : Constant  Value=TRUE  OutDataTypeStr=boolean
  True_VHAL_EPB1CSErr_flg : Constant  Value=TRUE  OutDataTypeStr=boolean
  True_VHAL_EPB1RCErr_flg : Constant  Value=TRUE  OutDataTypeStr=boolean
  True_VHAL_EPB1RC_enum : Constant  Value=TRUE  OutDataTypeStr=boolean
  True_VHAL_EPBCarWashMode_flg : Constant  Value=TRUE  OutDataTypeStr=boolean
  True_VHAL_EPBErrSta_enum : Constant  Value=TRUE  OutDataTypeStr=boolean
  True_VHAL_EPBExtApplyAvail_flg : Constant  Value=TRUE  OutDataTypeStr=boolean
  True_VHAL_EPBExtReleaseAvail_flg : Constant  Value=TRUE  OutDataTypeStr=boolean
  True_VHAL_EPBSta_enum : Constant  Value=TRUE  OutDataTypeStr=boolean
  slr1_{1..9} (9 alike) : BusSelector  OutputSignals=VINP_CANMsgValidEPB1_flg
  slr_VHAL_DOASta_flg : BusSelector  OutputSignals=VHAL_DOASta_flg
  slr_VHAL_EPB1CSErr_flg : BusSelector  OutputSignals=VHAL_EPB1CSErr_flg
  slr_VHAL_EPB1RCErr_flg : BusSelector  OutputSignals=VHAL_EPB1RCErr_flg
  slr_VHAL_EPB1RC_enum : BusSelector  OutputSignals=VHAL_EPB1RC_enum
  slr_VHAL_EPBCarWashMode_flg : BusSelector  OutputSignals=VHAL_EPBCarWashMode_flg
  slr_VHAL_EPBErrSta_enum : BusSelector  OutputSignals=VHAL_EPBErrSta_enum
  slr_VHAL_EPBExtApplyAvail_flg : BusSelector  OutputSignals=VHAL_EPBExtApplyAvail_flg
  slr_VHAL_EPBExtReleaseAvail_flg : BusSelector  OutputSignals=VHAL_EPBExtReleaseAvail_flg
  slr_VHAL_EPBSta_enum : BusSelector  OutputSignals=VHAL_EPBSta_enum
  VINP_EPB1CSErr_flg : Outport
  VINP_EPB1RCErr_flg : Outport  Port=2
  VINP_DOASta_flg : Outport  Port=3
  VINP_EPB1RC_enum : Outport  Port=4
  VINP_EPBCarWashMode_flg : Outport  Port=5
  VINP_EPBErrSta_enum : Outport  Port=6
  VINP_EPBExtApplyAvail_flg : Outport  Port=7
  VINP_EPBExtReleaseAvail_flg : Outport  Port=8
  VINP_EPBSta_enum : Outport  Port=9
  wires:
  BHAL_outputs/1 -> [BHAL_outputs]
  inp_CanValid_bus/1 -> [inp_CanValid_bus]
  [BHAL_outputs] -> slr_VHAL_EPB1CSErr_flg/1
  slr_VHAL_EPB1CSErr_flg/1 -> EPB1CSErr/1  "<VHAL_EPB1CSErr_flg>"
  True_VHAL_EPB1CSErr_flg/1 -> EPB1CSErr/2
  [inp_CanValid_bus] -> slr1_1/1
  slr1_1/1 -> EPB1CSErr/3  "<VINP_CANMsgValidEPB1_flg>"
  EPB1CSErr/1 -> VINP_EPB1CSErr_flg/1  "VINP_EPB1CSErr_flg"
  EPB1CSErr/2 -> Terminator_1/1
  [BHAL_outputs] -> slr_VHAL_EPB1RCErr_flg/1
  slr_VHAL_EPB1RCErr_flg/1 -> EPB1RCErr/1  "<VHAL_EPB1RCErr_flg>"
  True_VHAL_EPB1RCErr_flg/1 -> EPB1RCErr/2
  [inp_CanValid_bus] -> slr1_2/1
  slr1_2/1 -> EPB1RCErr/3  "<VINP_CANMsgValidEPB1_flg>"
  EPB1RCErr/1 -> VINP_EPB1RCErr_flg/1  "VINP_EPB1RCErr_flg"
  EPB1RCErr/2 -> Terminator_2/1
  [BHAL_outputs] -> slr_VHAL_DOASta_flg/1
  slr_VHAL_DOASta_flg/1 -> DOASta/1  "<VHAL_DOASta_flg>"
  True_VHAL_DOASta_flg/1 -> DOASta/2
  [inp_CanValid_bus] -> slr1_3/1
  slr1_3/1 -> DOASta/3  "<VINP_CANMsgValidEPB1_flg>"
  DOASta/1 -> VINP_DOASta_flg/1  "VINP_DOASta_flg"
  DOASta/2 -> Terminator_3/1
  [BHAL_outputs] -> slr_VHAL_EPB1RC_enum/1
  slr_VHAL_EPB1RC_enum/1 -> EPB1RC/1  "<VHAL_EPB1RC_enum>"
  True_VHAL_EPB1RC_enum/1 -> EPB1RC/2
  [inp_CanValid_bus] -> slr1_4/1
  slr1_4/1 -> EPB1RC/3  "<VINP_CANMsgValidEPB1_flg>"
  EPB1RC/1 -> VINP_EPB1RC_enum/1  "VINP_EPB1RC_enum"
  EPB1RC/2 -> Terminator_4/1
  [BHAL_outputs] -> slr_VHAL_EPBCarWashMode_flg/1
  slr_VHAL_EPBCarWashMode_flg/1 -> EPBCarWashMode/1  "<VHAL_EPBCarWashMode_flg>"
  True_VHAL_EPBCarWashMode_flg/1 -> EPBCarWashMode/2
  [inp_CanValid_bus] -> slr1_5/1
  slr1_5/1 -> EPBCarWashMode/3  "<VINP_CANMsgValidEPB1_flg>"
  EPBCarWashMode/1 -> VINP_EPBCarWashMode_flg/1  "VINP_EPBCarWashMode_flg"
  EPBCarWashMode/2 -> Terminator_5/1
  [BHAL_outputs] -> slr_VHAL_EPBErrSta_enum/1
  slr_VHAL_EPBErrSta_enum/1 -> EPBErrSta/1  "<VHAL_EPBErrSta_enum>"
  True_VHAL_EPBErrSta_enum/1 -> EPBErrSta/2
  [inp_CanValid_bus] -> slr1_6/1
  slr1_6/1 -> EPBErrSta/3  "<VINP_CANMsgValidEPB1_flg>"
  EPBErrSta/1 -> VINP_EPBErrSta_enum/1  "VINP_EPBErrSta_enum"
  EPBErrSta/2 -> Terminator_6/1
  [BHAL_outputs] -> slr_VHAL_EPBExtApplyAvail_flg/1
  slr_VHAL_EPBExtApplyAvail_flg/1 -> EPBExtApplyAvail/1  "<VHAL_EPBExtApplyAvail_flg>"
  True_VHAL_EPBExtApplyAvail_flg/1 -> EPBExtApplyAvail/2
  [inp_CanValid_bus] -> slr1_7/1
  slr1_7/1 -> EPBExtApplyAvail/3  "<VINP_CANMsgValidEPB1_flg>"
  EPBExtApplyAvail/1 -> VINP_EPBExtApplyAvail_flg/1  "VINP_EPBExtApplyAvail_flg"
  EPBExtApplyAvail/2 -> Terminator_7/1
  [BHAL_outputs] -> slr_VHAL_EPBExtReleaseAvail_flg/1
  slr_VHAL_EPBExtReleaseAvail_flg/1 -> EPBExtReleaseAvail/1  "<VHAL_EPBExtReleaseAvail_flg>"
  True_VHAL_EPBExtReleaseAvail_flg/1 -> EPBExtReleaseAvail/2
  [inp_CanValid_bus] -> slr1_8/1
  slr1_8/1 -> EPBExtReleaseAvail/3  "<VINP_CANMsgValidEPB1_flg>"
  EPBExtReleaseAvail/1 -> VINP_EPBExtReleaseAvail_flg/1  "VINP_EPBExtReleaseAvail_flg"
  EPBExtReleaseAvail/2 -> Terminator_8/1
  [BHAL_outputs] -> slr_VHAL_EPBSta_enum/1
  slr_VHAL_EPBSta_enum/1 -> EPBSta/1  "<VHAL_EPBSta_enum>"
  True_VHAL_EPBSta_enum/1 -> EPBSta/2
  [inp_CanValid_bus] -> slr1_9/1
  slr1_9/1 -> EPBSta/3  "<VINP_CANMsgValidEPB1_flg>"
  EPBSta/1 -> VINP_EPBSta_enum/1  "VINP_EPBSta_enum"
  EPBSta/2 -> Terminator_9/1
